simulink model "LKA_Lenkung_IPG_Horn"  (Simulink 7.4)
settings: Solver=ode4  StartTime=0.0  StopTime=tend-1  FixedStep=0.01  MaxStep=0.3  RelTol=1e-3
values from neighbouring files (symbols this model uses):
  epsL = block.ContStates.Data(2)    [lkaLaneTrackingMdl_SFcn.m]    (also in lkaPlot.m = ret.(fNameret{1}).epsL.value)
  P = P(1)    [LKA_Lenkung_CarMaker_DSR_kaskadiert_.m]    (also in LKA_Lenkung_CarMaker_DSR_kombiniert_algSynth_.m = tf(sysSingleTrackVisDSR); Lenkung_CarMaker_DSR_.m = tf(sysSteeringModel); lkaController_s.m = tf(sysSingleTrackVis); lkaLaneTracking.m = [obj.x(1);obj.y(1)] - xyCG_global)
  R = 10    [LKA_Lenkung_CarMaker_DSR_kombiniert_.m]    (also in lkaController2_t.m = 2; lkaController_t.m; ssMdl_EPS.m = 0.035)
  V = 3    [ssMdl_EPS.m]
  yL = block.ContStates.Data(1)    [lkaLaneTrackingMdl_SFcn.m]    (also in lkaPlot.m = ret.(fNameret{1}).yL.value)
undefined symbols (not defined in the file or in its folder): minreal
libraries: library x4, cstblocks x3
settings Model: Creator=Georg  LastModifiedBy=Georg

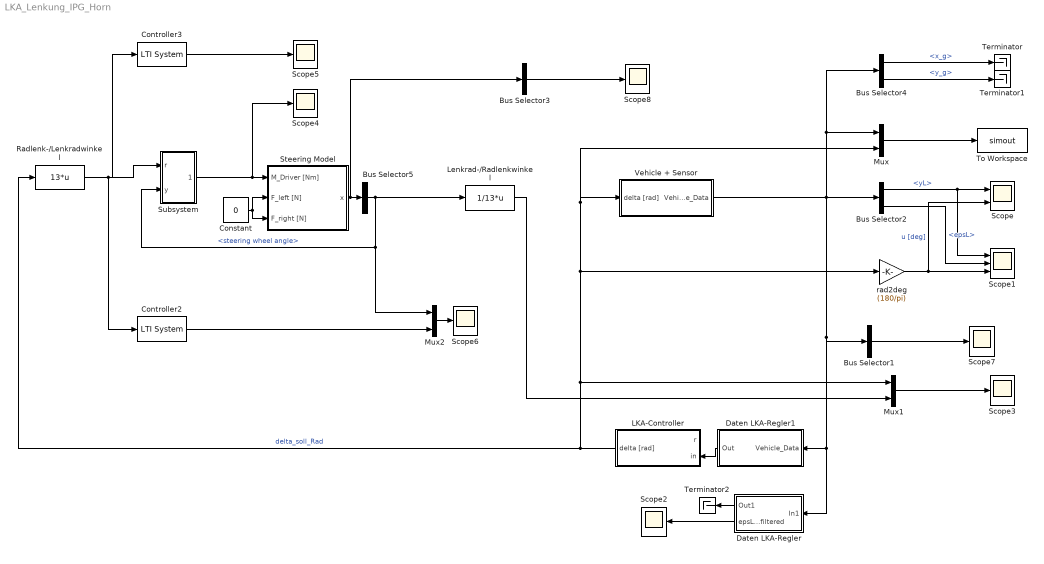
== system LKA_Lenkung_IPG_Horn ==
  Bus Selector1 : BusSelector  OutputSignals=Vehicle_State.s_yDot,Vehicle_State.psiDot  OutputAsBus=on
  Bus Selector2 : BusSelector  OutputSignals=Vehicle_Video_Sensor.yL,Vehicle_Video_Sensor.epsL
  Bus Selector3 : BusSelector  OutputSignals=steering wheel angle,steering wheel angle velocity  OutputAsBus=on
  Bus Selector4 : BusSelector  OutputSignals=Vehicle_State.x_g,Vehicle_State.y_g
  Bus Selector5 : BusSelector  OutputSignals=steering wheel angle
  Constant : Constant  Value=0  OutDataType=fixdt(1, 16)  OutScaling=2^0
  Controller2 : cstblocks/LTI System  SystemSampleTime=-1  sys=Tsoll  IC=[]
  Controller3 : cstblocks/LTI System  SystemSampleTime=-1  sys=minreal(V/(1+R*P(1)))  IC=[]
  Daten LKA-Regler : Subsystem  mask{sw_on_off=0, fg=40}
      mask prompts: sw_on_off "Filter On/Off"; fg "Grenzfrequenz"
      mask Display: disp(['Filter: ',num2str(sw_on_off)])
  Daten LKA-Regler1 : Subsystem  BlockChoice=yL/epsL geschätzt
      settings: AttributesFormatString=%<BlockChoice>  TemplateBlock=library/LKA-Sensorik/Daten LKA-Regler  MemberBlocks=yL Sensor / epsL Modell,yL/epsL Modell,yL/epsL Sensor
  LKA-Controller : Subsystem  BlockChoice=LQR_2int
      settings: AttributesFormatString=%<BlockChoice>  TemplateBlock=library/LKA-Controller/LKA-Controller  MemberBlocks=AlgSynth,FKL,LQR,LQR_2int,ZR,ZR_2int
  Lenkrad-/Radlenkwinkel : MATLABFcn  MATLABFcn=1/13*u
  Mux : Mux  Inputs=2
  Mux1 : Mux  Inputs=2
  Mux2 : Mux  Inputs=2
  Radlenk-/Lenkradwinkel : MATLABFcn  MATLABFcn=13*u
  Scope : Scope  NumInputPorts=2
      settings: TimeRange=20  YMin=-0.0125~0  YMax=0.0225~1.8
  Scope1 : Scope  NumInputPorts=3
      settings: TimeRange=20  YMin=-0.00175~0.01745~1.06  YMax=0.00225~0.0181~1.0875
  Scope{2..8} (7 alike) : Scope
      Scope2 settings: YMin=0.017122  YMax=0.0171335  SaveName=ScopeData2
      Scope3 settings: TimeRange=20  YMin=0  YMax=0.02  SaveName=ScopeData3
      Scope4 settings: YMin=0  YMax=0.00105  SaveName=ScopeData4
      Scope5 settings: YMin=0  YMax=0.019  SaveName=ScopeData6
      Scope6 settings: TimeRange=20  YMin=0.158  YMax=0.181  SaveName=ScopeData7
      Scope7 settings: TimeRange=20  YMin=-0.2  YMax=0.15  SaveName=ScopeData8
      Scope8 settings: TimeRange=20  YMin=-0.025  YMax=0.475  SaveName=ScopeData9
  Steering Model : Subsystem  BlockChoice=CarMaker DSR
      settings: AttributesFormatString=%<BlockChoice>  TemplateBlock=library/Steering Models/Steering Model  MemberBlocks=CarMaker DSR
  Subsystem : Subsystem
  Terminator : Terminator
  Terminator1 : Terminator
  Terminator2 : Terminator
  To Workspace : ToWorkspace  VariableName=simout  SampleTime=-1  SaveFormat=Structure With Time
  Vehicle + Sensor : Subsystem  BlockChoice=Einspurmodell + Rel.position mit Sensor
      settings: AttributesFormatString=%<BlockChoice>  TemplateBlock=library/Vehicle+Sensor/Vehicle + Sensor  MemberBlocks=Einspurmodell + Rel.position mit Sensor ,Einspurmodell mit Sensor
  "rad2deg " : Gain  Gain=(180/pi)  ParameterDataType=fixdt(1, 16)  ParameterScaling=2^0  OutDataType=fixdt(1, 16)  OutScaling=2^0
  wires:
  Bus Selector4/1 -> Terminator/1  "<x_g>"
  Bus Selector4/2 -> Terminator1/1  "<y_g>"
  LKA-Controller/1(delta [rad]) -> Mux1/1, "rad2deg "/1, Mux/2, Vehicle + Sensor/1(delta [rad]), Radlenk-/Lenkradwinkel/1  "delta_soll_Rad"
  Bus Selector2/1 -> Scope/1, Scope1/1  "<yL>"
  Mux/1 -> To Workspace/1
  Bus Selector2/2 -> Scope1/2  "<epsL>"
  "rad2deg "/1 -> Scope/2, Scope1/3  "u [deg]"
  Vehicle + Sensor/1(Vehicle_Data) -> Bus Selector2/1, Mux/1, Bus Selector4/1, Daten LKA-Regler/1(In1), Daten LKA-Regler1/1(Vehicle_Data), Bus Selector1/1
  Mux1/1 -> Scope3/1
  Daten LKA-Regler/2(epsL (un)filtered) -> Scope2/1
  Subsystem/1(Out1) -> Scope4/1, Steering Model/1(M_Driver [Nm])
  Mux2/1 -> Scope6/1
  Controller2/1 -> Mux2/2
  Steering Model/1(x) -> Bus Selector5/1, Bus Selector3/1
  Bus Selector5/1 -> Lenkrad-/Radlenkwinkel/1, Mux2/1, Subsystem/2(y)  "<steering wheel angle>"
  Controller3/1 -> Scope5/1
  Radlenk-/Lenkradwinkel/1 -> Controller2/1, Controller3/1, Subsystem/1(r)
  Lenkrad-/Radlenkwinkel/1 -> Mux1/2
  Constant/1 -> Steering Model/2(F_left [N]), Steering Model/3(F_right [N])
  Bus Selector1/1 -> Scope7/1
  Bus Selector3/1 -> Scope8/1
  Daten LKA-Regler/1(Out1) -> Terminator2/1
  Daten LKA-Regler1/1(Out) -> LKA-Controller/2(in)

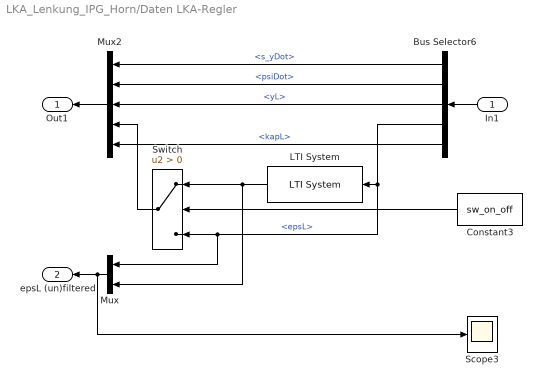
== system LKA_Lenkung_IPG_Horn/Daten LKA-Regler ==
  In1 : Inport
  Bus Selector6 : BusSelector  OutputSignals=Vehicle_State.s_yDot,Vehicle_State.psiDot,Vehicle_Video_Sensor.yL,Vehicle_Video_Sensor.epsL,Vehicle_Video_Sensor.kapL
  Constant3 : Constant  Value=sw_on_off  OutDataType=fixdt(1, 16)  OutScaling=2^0
  LTI System : cstblocks/LTI System  SystemSampleTime=-1  sys=zpk([],[-fg],fg)  IC=[]
  Mux : Mux  Inputs=2
  Mux2 : Mux  Inputs=5
  Scope3 : Scope
      settings: TimeRange=20  YMin=0.0102  YMax=0.0112  SaveName=ScopeData5
  Switch : Switch  Criteria=u2 > Threshold  OutDataType=fixdt(1, 16)  OutScaling=2^0
  Out1 : Outport
  epsL (un)filtered : Outport  Port=2
  wires:
  In1/1 -> Bus Selector6/1
  Mux2/1 -> Out1/1
  Bus Selector6/4 -> LTI System/1, Switch/3, Mux/1  "<epsL>"
  LTI System/1 -> Switch/1, Mux/2
  Constant3/1 -> Switch/2
  Mux/1 -> epsL (un)filtered/1, Scope3/1
  Bus Selector6/1 -> Mux2/1  "<s_yDot>"
  Bus Selector6/2 -> Mux2/2  "<psiDot>"
  Bus Selector6/3 -> Mux2/3  "<yL>"
  Switch/1 -> Mux2/4
  Bus Selector6/5 -> Mux2/5  "<kapL>"

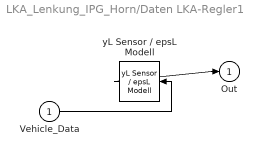
== system LKA_Lenkung_IPG_Horn/Daten LKA-Regler1 ==
  Vehicle_Data : Inport
  yL Sensor / epsL Modell : library/LKA-Sensorik/yL Sensor // epsL Modell  SystemSampleTime=-1
  Out : Outport
  wires:
  yL Sensor / epsL Modell/1 -> Out/1
  Vehicle_Data/1 -> yL Sensor / epsL Modell/1

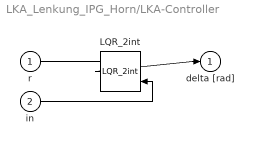
== system LKA_Lenkung_IPG_Horn/LKA-Controller ==
  r : Inport
  in : Inport  Port=2
  LQR_2int : library/LKA-Controller/LQR_2int  SystemSampleTime=-1
  delta [rad] : Outport
  wires:
  r/1 -> LQR_2int/1
  in/1 -> LQR_2int/2
  LQR_2int/1 -> delta [rad]/1

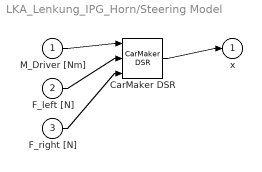
== system LKA_Lenkung_IPG_Horn/Steering Model ==
  M_Driver [Nm] : Inport
  F_left [N] : Inport  Port=2
  F_right [N] : Inport  Port=3
  CarMaker DSR : library/Steering Models/CarMaker DSR  SystemSampleTime=-1
  x : Outport
  wires:
  M_Driver [Nm]/1 -> CarMaker DSR/1
  F_left [N]/1 -> CarMaker DSR/2
  F_right [N]/1 -> CarMaker DSR/3
  CarMaker DSR/1 -> x/1

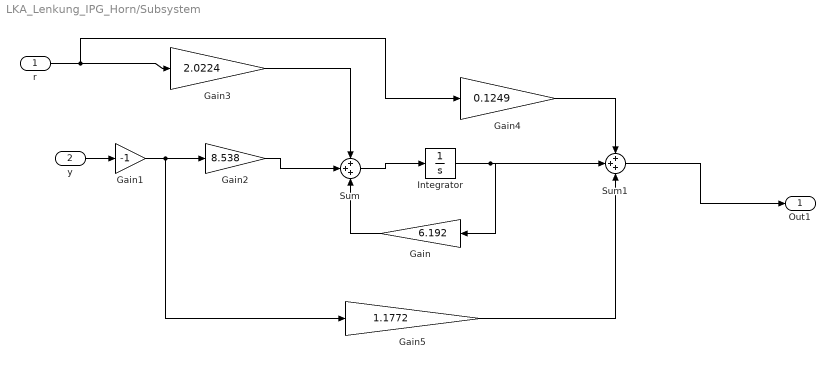
== system LKA_Lenkung_IPG_Horn/Subsystem ==
  r : Inport
  y : Inport  Port=2
  Gain : Gain  Gain=6.192  ParameterDataType=fixdt(1, 16)  ParameterScaling=2^0  OutDataType=fixdt(1, 16)  OutScaling=2^0
  Gain1 : Gain  Gain=-1  ParameterDataType=fixdt(1, 16)  ParameterScaling=2^0  OutDataType=fixdt(1, 16)  OutScaling=2^0
  Gain2 : Gain  Gain=8.538  ParameterDataType=fixdt(1, 16)  ParameterScaling=2^0  OutDataType=fixdt(1, 16)  OutScaling=2^0
  Gain3 : Gain  Gain=2.0224  ParameterDataType=fixdt(1, 16)  ParameterScaling=2^0  OutDataType=fixdt(1, 16)  OutScaling=2^0
  Gain4 : Gain  Gain=0.1249  ParameterDataType=fixdt(1, 16)  ParameterScaling=2^0  OutDataType=fixdt(1, 16)  OutScaling=2^0
  Gain5 : Gain  Gain=1.1772  ParameterDataType=fixdt(1, 16)  ParameterScaling=2^0  OutDataType=fixdt(1, 16)  OutScaling=2^0
  Integrator : Integrator
  Sum : Sum  Inputs=+++  OutDataType=fixdt(1, 16)  OutScaling=2^0
  Sum1 : Sum  Inputs=+++  OutDataType=fixdt(1, 16)  OutScaling=2^0
  Out1 : Outport
  wires:
  Gain/1 -> Sum/3
  Sum/1 -> Integrator/1
  y/1 -> Gain1/1
  Gain1/1 -> Gain2/1, Gain5/1
  Gain2/1 -> Sum/2
  r/1 -> Gain3/1, Gain4/1
  Gain3/1 -> Sum/1
  Integrator/1 -> Gain/1, Sum1/2
  Gain4/1 -> Sum1/1
  Gain5/1 -> Sum1/3
  Sum1/1 -> Out1/1

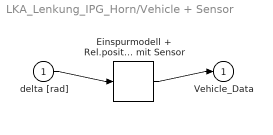
== system LKA_Lenkung_IPG_Horn/Vehicle + Sensor ==
  delta [rad] : Inport
  "Einspurmodell + Rel.position mit Sensor " : library/Vehicle+Sensor/Einspurmodell + Rel.position mit Sensor   SystemSampleTime=-1
  Vehicle_Data : Outport
  wires:
  delta [rad]/1 -> "Einspurmodell + Rel.position mit Sensor "/1
  "Einspurmodell + Rel.position mit Sensor "/1 -> Vehicle_Data/1
